simulink model "Coordinate Simulation"  (R2021a)
settings: Solver=VariableStepAuto  StartTime=0.0  StopTime=10.0  RelTol=1e-3
settings Model: Creator=alber  LastModifiedBy=alber

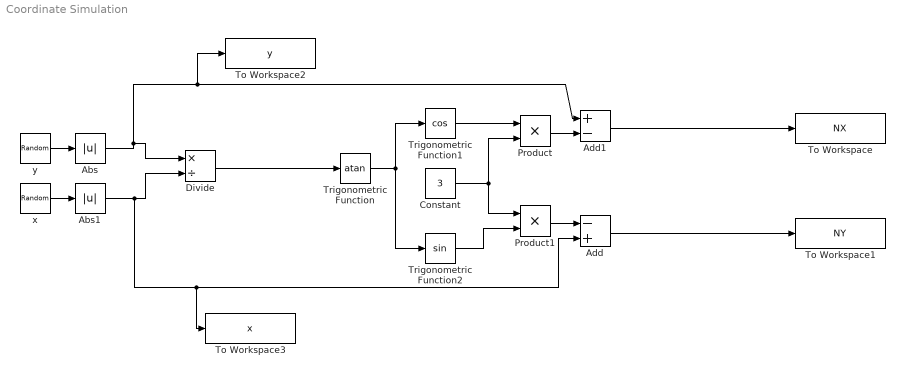
== system Coordinate Simulation ==
  Abs : Abs
  Abs1 : Abs
  Add : Sum  Inputs=-+
  Add1 : Sum  Inputs=+-
  Constant : Constant  Value=3
  Divide : Product  Inputs=*/
  Product : Product
  Product1 : Product
  To Workspace : ToWorkspace  VariableName=NX  SampleTime=-1
      settings: Save2DSignal=2-D array (concatenate along first dimension)
  To Workspace1 : ToWorkspace  VariableName=NY  SampleTime=-1
      settings: Save2DSignal=2-D array (concatenate along first dimension)
  To Workspace2 : ToWorkspace  VariableName=y  SampleTime=-1
      settings: Save2DSignal=2-D array (concatenate along first dimension)
  To Workspace3 : ToWorkspace  VariableName=x  SampleTime=-1
      settings: Save2DSignal=2-D array (concatenate along first dimension)
  Trigonometric Function : Trigonometry  Operator=atan
  Trigonometric Function1 : Trigonometry  Operator=cos
  Trigonometric Function2 : Trigonometry
  x : RandomNumber  Mean=5  Variance=10  Seed=5  SampleTime=0.1
  y : RandomNumber  Mean=5  Variance=10  Seed=1  SampleTime=0.1
  wires:
  x/1 -> Abs1/1
  y/1 -> Abs/1
  Divide/1 -> Trigonometric Function/1
  Trigonometric Function/1 -> Trigonometric Function1/1, Trigonometric Function2/1
  Trigonometric Function2/1 -> Product1/2
  Constant/1 -> Product/2, Product1/1
  Trigonometric Function1/1 -> Product/1
  Product1/1 -> Add/1
  Product/1 -> Add1/2
  Add1/1 -> To Workspace/1
  Add/1 -> To Workspace1/1
  Abs/1 -> To Workspace2/1, Add1/1, Divide/1
  Abs1/1 -> To Workspace3/1, Add/2, Divide/2
